simulink model "CHW1_Q11_Simulink"  (R2021b)
settings: Solver=VariableStepAuto  StartTime=0.0  StopTime=16.0  RelTol=1e-3
settings Model: Creator=A  LastModifiedBy=Matin

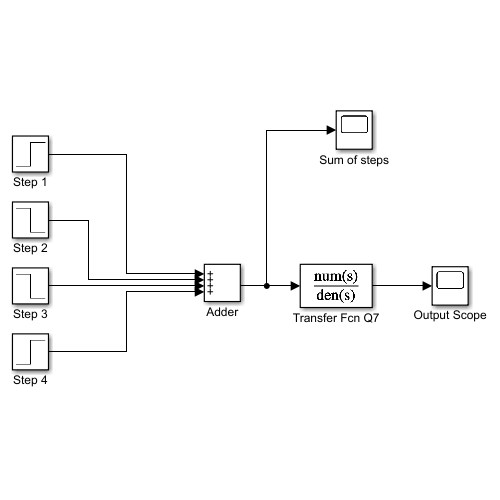
[thumbnail: Simulink's stored preview of the top-level diagram]
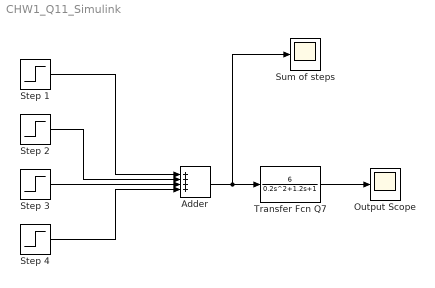
== system CHW1_Q11_Simulink ==
  Adder : Sum  Inputs=++++
  Output Scope : Scope
  Step 1 : Step  Time=2  After=2  SampleTime=0
  Step 2 : Step  Time=6  After=-2  SampleTime=0
  Step 3 : Step  Time=8  After=-1  SampleTime=0
  Step 4 : Step  Time=12  SampleTime=0
  Sum of steps : Scope
  Transfer Fcn Q7 : TransferFcn  Numerator=[0 0 6]  Denominator=[0.2 1.2 1]
  wires:
  Step 2/1 -> Adder/2
  Step 1/1 -> Adder/1
  Step 3/1 -> Adder/3
  Step 4/1 -> Adder/4
  Adder/1 -> Sum of steps/1, Transfer Fcn Q7/1
  Transfer Fcn Q7/1 -> Output Scope/1
